simulink library "dspswit3"  (Simulink 8.0)
settings: Solver=ode45  SolverMode=SingleTasking  StartTime=0.0  StopTime=10.0  RelTol=1e-3
values from neighbouring files (symbols this model uses):
  D = D + B    [rebuffer_delay.m]
undefined symbols (not defined in the file or in its folder): High, Low
libraries: dspsigattribs x4, dspsigops x3, dspsrcs4 x1, dspswit3 x1
settings Model: RequirementInfo=9  Creator=don  LastModifiedBy=lij  ExtModeAutoUpdateStatusClock=off

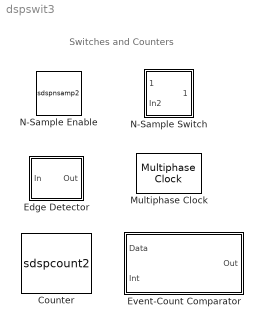
== system dspswit3 ==
  note: Switches and Counters
  Counter : S-Function  FunctionName=sdspcount2  Parameters=Direction, CountEvent, CounterSize, MaxCount, InitialCount, Output, HitValue, ResetInput, SamplesPerFrame, Ts, CntDtype, HitDtype  EnableBusSupport=off  mask(Counter){Direction=Up, CountEvent=Rising edge, CounterSize=User defined, MaxCount=255, InitialCount=0, Output=Count and Hit, HitValue=32, ResetInput=on, SamplesPerFrame=1, Ts=1, CntDtype=double, HitDtype=Logical}
      mask prompts: Direction "Count direction:"; CountEvent "Count event:"; CounterSize "Counter size:"; MaxCount "Maximum count:"; InitialCount "Initial count:"; HitValue "Hit values:"; ResetInput "Reset input"; SamplesPerFrame "Samples per output frame"; Ts "Sample time:"; CntDtype "Count data type:"; HitDtype "Hit data type:"
      mask help: Count up or down through a specified range of numbers. If you set the 'Count event' parameter to 'Free running', the block counts at a constant time interval. Otherwise, the block increments or decrements the counter each time a trigger event occurs at the Inc/Dec input port.
      mask init:
      | [str] = dspblkcount2('icon');
      | set_param(gcbh, 'MaskDisplay', str);
      mask Help: eval('blocksethelp');
      mask StyleString: popup(Up|Down),popup(Rising edge|Falling edge|Either edge|Non-zero sample|Free running),popup(8 bits|16 bits|32 bits|User defined|Specify via input port),edit,edit,popup(Count|Hit|Count and Hit),edit,checkbox,edit,edit,popup(double|single|int8|uint8|int16|uint16|int32|uint32),popup(Logical|Boolean)
      mask CallbackString: |dspblkcount2|dspblkcount2|||dspblkcount2||dspblkcount2|||dspblkcount2|
      mask Display: disp('Count\nUp');port_label('input',1,'Inc');port_label('input',2,'Rst');port_label('output',1,'Cnt');port_label('output',2,'Hit');
  Edge Detector : Subsystem  mask(Edge Detector){InputProcessing=Columns as channels (frame based)}
      mask prompts: InputProcessing "Input processing:"
      mask help: Output a unity amplitude pulse for one sample period in response to a transition from zero to a nonzero value.
      mask init:
      | [x,y] = dspblkedetect2('icon');
      | dspblkedetect2('init', gcbh, gcb);
      mask Help: eval('blocksethelp');
      mask StyleString: popup(Columns as channels (frame based)|Elements as channels (sample based)|Inherited (this choice will be removed - see release notes))
      mask Display: plot(x,y)
  Event-Count Comparator : Subsystem  mask(Event-Count Comparator){Threshold=10}
      mask prompts: Threshold "Event threshold:"
      mask help: Output is true if the number of nonzero inputs over time equals or exceeds the 'Event threshold' during the enable interval. A nonzero input on the interval port (Int) enables the block to begin counting and resets the output. Inputs must be discrete-time scalars.
      mask init:
      | ThresholdValue = get_param(gcbh, 'Threshold');
      | dtcBlk = [gcb '/Data Type Conversion'];
      | if isempty(Threshold)
      |  s=ThresholdValue;
      | 	set_param(dtcBlk,'DataType','uint8');
      | else
      | 	dblThresh = double(Threshold);
      | 	s=num2str(dblThresh);
      | 	if (dblThresh <= 255)
      |     	set_param(dtcBlk,'DataType','uint8');
      | 	elseif (dblThresh <= 65535)
      |     	set_param(dtcBlk,'DataType','uint16');
      | 	else
      |     	set_param(dtcBlk,'DataType','uint32');
      | 	end
      | end
      mask Help: eval('blocksethelp');
      mask Display:
      | disp('Event-Count\nComparator')
      | text(0.95,0.1,['Thresh:' s],'horiz','right')
  Multiphase Clock : dspsrcs4/Multiphase Clock  ClkFreq=1  NumPhases=4  StartPhase=1  DutyCycle=3  ActiveLevel=High (1)  DataType=Logical
  N-Sample Enable : S-Function  FunctionName=sdspnsamp2  Parameters=TriggerTypeo, N, Ts, ActiveLevel,DataType,reset  EnableBusSupport=off  mask(N-Sample Enable){N=8, ActiveLevel=High (1), reset=off, TriggerType=Rising edge, Ts=1, DataType=Logical}
      mask prompts: N "Trigger count, N:"; ActiveLevel "Active level:"; reset "Reset input"; TriggerType "Trigger type:"; Ts "Sample time:"; DataType "Output data type:"
      mask help: Transition from inactive to active after the first N samples.
      mask init:
      | NValue = get_param(gcbh, 'N');
      | N = double(N);
      | [s,x,y, p] = dspblknsample('icon', N, NValue);
      | TriggerTypeo = dspblknsample('update', TriggerType);
      mask Help: eval('blocksethelp');
      mask StyleString: edit,popup(High (1)|Low (0)),checkbox,popup(Rising edge|Falling edge|Either edge|Non-zero sample),edit,popup(Logical|Boolean)
      mask CallbackString: ||dspblknsample|dspblknsample||
      mask Display:
      | plot(x,y);
      | text(1, 0.05, s,'horiz','right','vert','base');
      | port_label(p.side,p.port,p.label);
  N-Sample Switch : Subsystem  mask(N-Sample Switch){N=8, reset=off, TriggerType=Rising edge, Ts=0.1}
      mask prompts: N "Switch count, N:"; reset "Reset input"; TriggerType "Trigger type:"; Ts "Sample time:"
      mask help: Output N samples from the top port. Thereafter, output samples from the bottom port.
      mask init:
      | NValue = get_param(gcbh, 'N');
      | N = double(N);
      | [s, x,y] = dspblknswit('icon',N,NValue);
      | dspblknswit('update');
      mask Help: eval('blocksethelp');
      mask StyleString: edit,checkbox,popup(Rising edge|Falling edge|Either edge|Non-zero sample),edit
      mask CallbackString: |dspblknswit||
      mask Display:
      | plot(x,y);
      | text(1, 0.05, s,'horiz','right','vert','base');

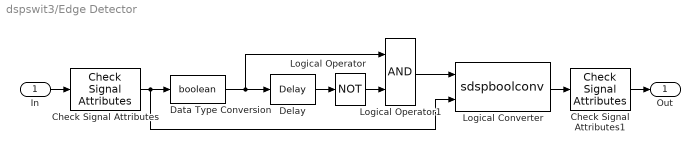
== system dspswit3/Edge Detector ==
  In : Inport
  Check Signal Attributes : dspsigattribs/Check Signal Attributes  SystemSampleTime=-1  SigAttribCheckMethod=Matches attributes exactly  Complexity=Ignore  Frame=Ignore  DimsCheckMethod=Ignore  Dimensions=1-D  DatatypeCheckMethod=Is...  DatatypeGeneral=Enumerated  DtypeFloatSpecific=Any floating-point  DtypeFixedSpecific=Any fixed-point  DtypeIntSpecific=Any integer  SampleMode=Ignore
  Check Signal Attributes1 : dspsigattribs/Check Signal Attributes  SystemSampleTime=-1  SigAttribCheckMethod=Matches attributes exactly  Complexity=Ignore  Frame=Ignore  DimsCheckMethod=Ignore  Dimensions=1-D  DatatypeCheckMethod=Is...  DatatypeGeneral=Enumerated  DtypeFloatSpecific=Any floating-point  DtypeFixedSpecific=Any fixed-point  DtypeIntSpecific=Any integer  SampleMode=Ignore
  Data Type Conversion : DataTypeConversion  OutDataTypeStr=boolean  SaturateOnIntegerOverflow=on  RndMeth=Zero
  Delay : dspsigops/Delay  InputProcessing=Columns as channels (frame based)  dly_unit=Samples  delay=1  ic_detail=on  dif_ic_for_ch=off  dif_ic_for_dly=off  ic=1  reset_popup=None
  Logical Operator : Logic  Operator=NOT  Inputs=1
  Logical Operator1 : Logic
  Logical Converter : S-Function  FunctionName=sdspboolconv  EnableBusSupport=off
      mask Display:
      | disp('Logical\nConverter');
      | 
      | 
      | 
      | 
      | 
      | port_label('input',1, 'In');
      | 
      | 
      | 
      | 
      | 
      | port_label('input',2, 'Ref');
  Out : Outport  InitialOutput=0
  wires:
  Logical Operator1/1 -> Logical Converter/1
  Logical Operator/1 -> Logical Operator1/2
  Data Type Conversion/1 -> Logical Operator1/1, Delay/1
  Delay/1 -> Logical Operator/1
  In/1 -> Check Signal Attributes/1
  Logical Converter/1 -> Check Signal Attributes1/1
  Check Signal Attributes/1 -> Logical Converter/2, Data Type Conversion/1
  Check Signal Attributes1/1 -> Out/1

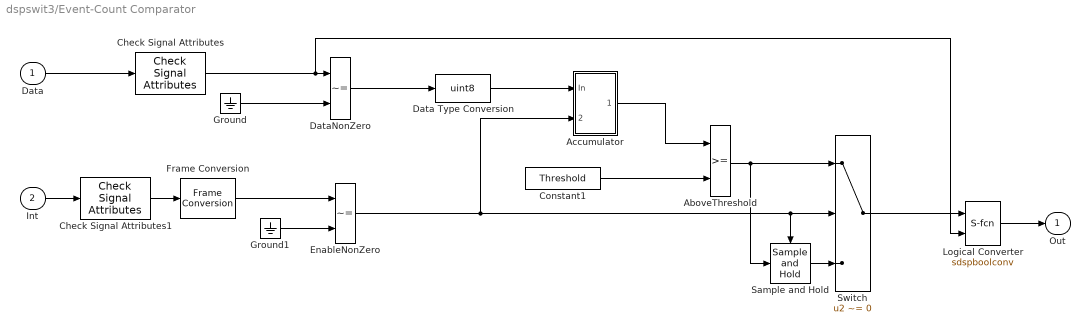
== system dspswit3/Event-Count Comparator ==
  Data : Inport
  Int : Inport  Port=2
  AboveThreshold : RelationalOperator  OutDataTypeStr=boolean  InputSameDT=on
  Accumulator : Subsystem
  Check Signal Attributes : dspsigattribs/Check Signal Attributes  SystemSampleTime=-1  SigAttribCheckMethod=Does not match attributes exactly  Complexity=Ignore  Frame=Ignore  DimsCheckMethod=Is...  Dimensions=Scalar (1-D or 2-D)  DatatypeCheckMethod=Is not...  DatatypeGeneral=Enumerated  DtypeFloatSpecific=Any floating-point  DtypeFixedSpecific=Any fixed-point  DtypeIntSpecific=Any integer  SampleMode=Discrete
  Check Signal Attributes1 : dspsigattribs/Check Signal Attributes  SystemSampleTime=-1  SigAttribCheckMethod=Does not match attributes exactly  Complexity=Ignore  Frame=Ignore  DimsCheckMethod=Is...  Dimensions=Scalar (1-D or 2-D)  DatatypeCheckMethod=Is not...  DatatypeGeneral=Enumerated  DtypeFloatSpecific=Any floating-point  DtypeFixedSpecific=Any fixed-point  DtypeIntSpecific=Any integer  SampleMode=Discrete
  Constant1 : Constant  Value=Threshold  OutDataTypeStr=Inherit: Inherit via back propagation
  Data Type Conversion : DataTypeConversion  OutDataTypeStr=uint8  RndMeth=Zero
  DataNonZero : RelationalOperator  Operator=~=  OutDataTypeStr=boolean  InputSameDT=on
  EnableNonZero : RelationalOperator  Operator=~=  OutDataTypeStr=boolean  InputSameDT=on
  Frame Conversion : FrameConversion  OutFrame=Sample-based
  Ground : Ground
  Ground1 : Ground
  Logical Converter : S-Function  FunctionName=sdspboolconv  EnableBusSupport=off
      mask Type: Logical Converter
      mask Display:
      | port_label('input',1, 'In');
      | 
      | port_label('input',2, 'Ref');
  Sample and Hold : dspsigops/Sample and Hold  SystemSampleTime=-1  trig=Falling edge  initCond=0  latchinput=off
  Switch : Switch  Criteria=u2 ~= 0  Threshold=1  InputSameDT=on
  Out : Outport
  wires:
  Accumulator/1(Acc) -> AboveThreshold/1
  Data Type Conversion/1 -> Accumulator/1(In)
  DataNonZero/1 -> Data Type Conversion/1
  Logical Converter/1 -> Out/1
  Switch/1 -> Logical Converter/1
  EnableNonZero/1 -> Accumulator/2(Rst), Sample and Hold/Trigger, Switch/2
  Check Signal Attributes1/1 -> Frame Conversion/1
  Int/1 -> Check Signal Attributes1/1
  Constant1/1 -> AboveThreshold/2
  Check Signal Attributes/1 -> Logical Converter/2, DataNonZero/1
  Data/1 -> Check Signal Attributes/1
  AboveThreshold/1 -> Switch/1, Sample and Hold/1
  Sample and Hold/1 -> Switch/3
  Ground/1 -> DataNonZero/2
  Ground1/1 -> EnableNonZero/2
  Frame Conversion/1 -> EnableNonZero/1

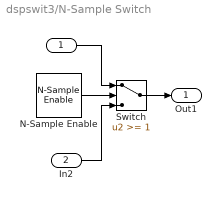
== system dspswit3/N-Sample Switch ==
  " " : Inport
  In2 : Inport  Port=2
  N-Sample Enable : dspswit3/N-Sample Enable  N=N  ActiveLevel=Low (0)  reset=off  TriggerType=Rising edge  Ts=Ts  DataType=Boolean
  Switch : Switch  Threshold=1  InputSameDT=on
  Out1 : Outport
  wires:
  N-Sample Enable/1 -> Switch/2
  Switch/1 -> Out1/1
  " "/1 -> Switch/1
  In2/1 -> Switch/3

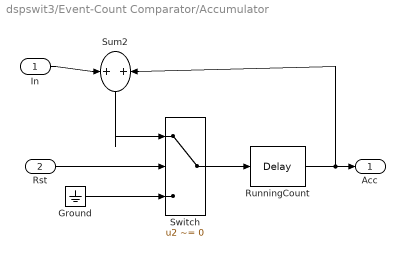
== system dspswit3/Event-Count Comparator/Accumulator ==
  In : Inport
  Rst : Inport  Port=2
  Ground : Ground
  RunningCount : dspsigops/Delay  InputProcessing=Columns as channels (frame based)  dly_unit=Samples  delay=1  ic_detail=off  dif_ic_for_ch=off  dif_ic_for_dly=off  ic=0  reset_popup=None
  Sum2 : Sum  Inputs=+|+  SaturateOnIntegerOverflow=on  InputSameDT=on  OutDataTypeStr=Inherit: Same as first input
  Switch : Switch  Criteria=u2 ~= 0  Threshold=1  ZeroCross=off
  Acc : Outport
  wires:
  In/1 -> Sum2/1
  Rst/1 -> Switch/2
  RunningCount/1 -> Acc/1, Sum2/2
  Switch/1 -> RunningCount/1
  Sum2/1 -> Switch/1
  Ground/1 -> Switch/3
